simulink library "MotorControlLibrary"  (R2025b)
settings: Solver=VariableStepAuto  StartTime=0.0  StopTime=10.0  RelTol=1e-3
libraries: $bdroot x5
settings Model: Creator=tka008729  LastModifiedBy=tka008729

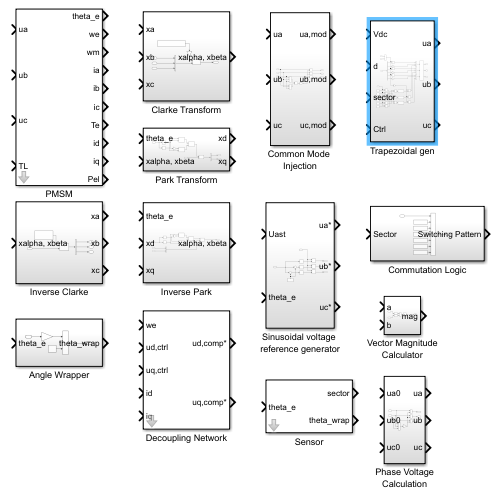
[thumbnail: Simulink's stored preview of the top-level diagram]
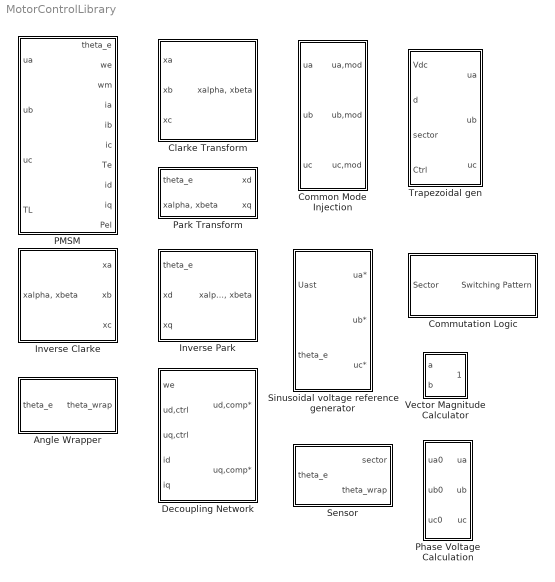
== system MotorControlLibrary ==
  Angle Wrapper : Subsystem
  Clarke Transform : Subsystem
  Common Mode Injection : Subsystem
  Commutation Logic : Subsystem
  Decoupling Network : Subsystem  mask(FOC Decoupling Network){Ls=0.000018, psi_PM=0.0021653734}
      mask prompts: Ls "Direct- and quadrute-axis inductances [Ls]"; psi_PM "Permanent magnet flux linkage [psi_PM]"
      mask help: Decouples direct- and quadrute-axis voltage components from eachother. Uses feedforward compensation. Relevant at higher speeds.
  Inverse Clarke : Subsystem
  Inverse Park : Subsystem
  PMSM : Subsystem  mask(PMSM){Rs=0.02125, Ls=0.000018, psi_PM=0.0021653734, p=14, J=0.0011, B=0.001}
      mask prompts: Rs "Phase resistance [Rs]"; Ls "Direct- and  quadrature-axis inductances [Ls]"; psi_PM "Permanent magnet flux linkage [psi_PM]"; p "Pole pairs [p]"; J "Moment of inertia [J]"; B "viscous friction coefficient [B]"
      mask help: Mathematical model of a non-salient permanent magnet synchronous motor (PMSM).
  Park Transform : Subsystem
  Phase Voltage Calculation : Subsystem
  Sensor : Subsystem  mask(Sector Sensor){phi_e=0}
      mask prompts: phi_e "Electrical angle offset [phi_e]"
      mask help: Converts continueous electrical angle in six-step control sector information.
  Sinusoidal voltage reference generator : Subsystem
  Trapezoidal gen : Subsystem
  Vector Magnitude Calculator : Subsystem

== system MotorControlLibrary/Angle Wrapper ==
  theta_e : Inport
  Constant : Constant  Value=360
  Gain6 : Gain  Gain=180/pi
  Math Function : Math  Operator=mod
  theta_wrap : Outport
  wires:
  Constant/1 -> Math Function/2
  Gain6/1 -> Math Function/1  "theta_deg"
  theta_e/1 -> Gain6/1
  Math Function/1 -> theta_wrap/1  "theta_wrap"

== system MotorControlLibrary/Clarke Transform ==
  xa : Inport
  xb : Inport  Port=2
  xc : Inport  Port=3
  Constant : Constant  Value=[1 -1/2 -1/2; 0 sqrt(3)/2 -sqrt(3)/2]
  Gain2 : Gain  Gain=2/3
  Mux : Mux  Inputs=3
  Product : Product  Multiplication=Matrix(*)
  "xalpha, xbeta" : Outport
  wires:
  xa/1 -> Mux/1
  xc/1 -> Mux/3
  Product/1 -> "xalpha, xbeta"/1
  Mux/1 -> Product/2
  Constant/1 -> Gain2/1
  xb/1 -> Mux/2
  Gain2/1 -> Product/1

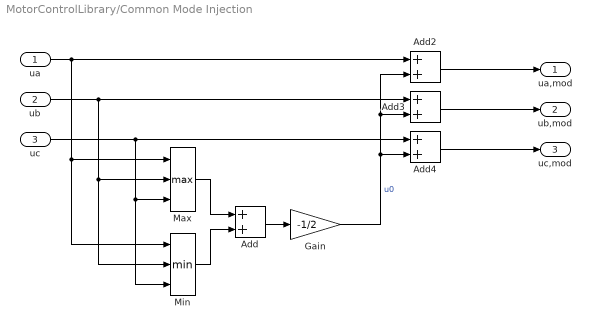
== system MotorControlLibrary/Common Mode Injection ==
  ua : Inport
  ub : Inport  Port=2
  uc : Inport  Port=3
  Add{,2..4} (4 alike) : Sum
  Gain : Gain  Gain=-1/2
  Max : MinMax  Function=max  Inputs=3
  Min : MinMax  Inputs=3
  ua,mod : Outport
  ub,mod : Outport  Port=2
  uc,mod : Outport  Port=3
  wires:
  Add2/1 -> ua,mod/1
  Add3/1 -> ub,mod/1
  Min/1 -> Add/2
  Add4/1 -> uc,mod/1
  Add/1 -> Gain/1
  Gain/1 -> Add2/2, Add3/2, Add4/2  "u0"
  ub/1 -> Max/2, Min/2, Add3/1
  Max/1 -> Add/1
  uc/1 -> Max/3, Min/3, Add4/1
  ua/1 -> Min/1, Max/1, Add2/1

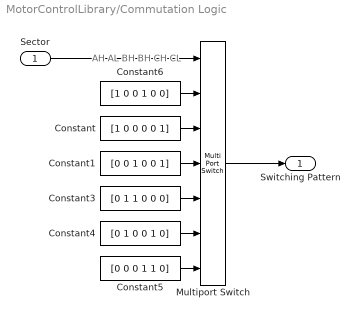
== system MotorControlLibrary/Commutation Logic ==
  note: AH AL BH BH CH CL
  Sector : Inport
  Constant : Constant  Value=[1 0 0 0 0 1]
  Constant1 : Constant  Value=[0 0 1 0 0 1]
  Constant3 : Constant  Value=[0 1 1 0 0 0]
  Constant4 : Constant  Value=[0 1 0 0 1 0]
  Constant5 : Constant  Value=[0 0 0 1 1 0]
  Constant6 : Constant  Value=[1 0 0 1 0 0]
  Multiport Switch : MultiPortSwitch  Inputs=6  DiagnosticForDefault=None  SaturateOnIntegerOverflow=off  InputSameDT=off
  Switching Pattern : Outport
  wires:
  Sector/1 -> Multiport Switch/1
  Multiport Switch/1 -> Switching Pattern/1
  Constant6/1 -> Multiport Switch/2
  Constant/1 -> Multiport Switch/3
  Constant1/1 -> Multiport Switch/4
  Constant3/1 -> Multiport Switch/5
  Constant5/1 -> Multiport Switch/7
  Constant4/1 -> Multiport Switch/6

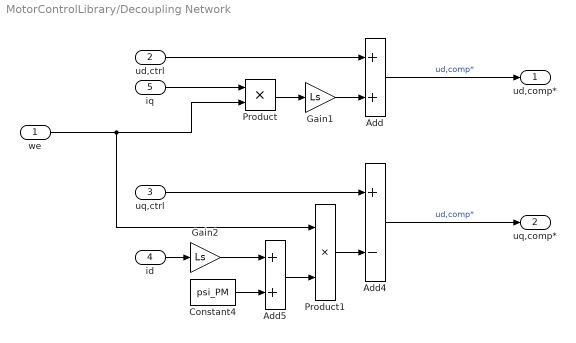
== system MotorControlLibrary/Decoupling Network ==
  we : Inport
  ud,ctrl : Inport  Port=2
  uq,ctrl : Inport  Port=3
  id : Inport  Port=4
  iq : Inport  Port=5
  Add : Sum
  Add4 : Sum  Inputs=+-
  Add5 : Sum
  Constant4 : Constant  Value=psi_PM
  Gain1 : Gain  Gain=Ls
  Gain2 : Gain  Gain=Ls
  Product : Product
  Product1 : Product
  ud,comp* : Outport
  uq,comp* : Outport  Port=2
  wires:
  iq/1 -> Product/1
  Product1/1 -> Add4/2
  Add5/1 -> Product1/2
  Constant4/1 -> Add5/2
  Gain2/1 -> Add5/1
  Add4/1 -> uq,comp*/1  "ud,comp*"
  Product/1 -> Gain1/1
  Gain1/1 -> Add/2
  ud,ctrl/1 -> Add/1
  id/1 -> Gain2/1
  Add/1 -> ud,comp*/1  "ud,comp*"
  we/1 -> Product1/1, Product/2
  uq,ctrl/1 -> Add4/1

== system MotorControlLibrary/Inverse Clarke ==
  "xalpha, xbeta" : Inport
  Constant1 : Constant  Value=[1 0; -1/2 sqrt(3)/2; -1/2 -sqrt(3)/2]
  Demux1 : Demux  Outputs=3
  Matrix Multiply : Product  Multiplication=Matrix(*)
  xa : Outport
  xb : Outport  Port=2
  xc : Outport  Port=3
  wires:
  Matrix Multiply/1 -> Demux1/1
  Constant1/1 -> Matrix Multiply/1
  Demux1/2 -> xb/1
  Demux1/3 -> xc/1
  Demux1/1 -> xa/1
  "xalpha, xbeta"/1 -> Matrix Multiply/2

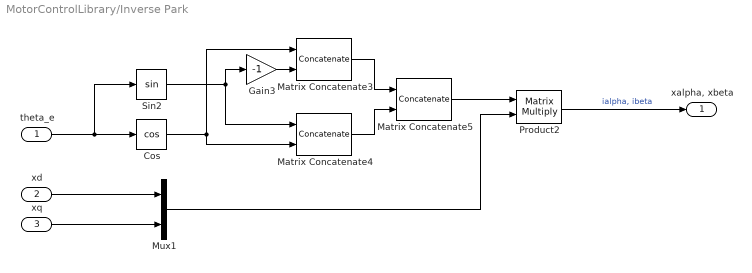
== system MotorControlLibrary/Inverse Park ==
  theta_e : Inport
  xd : Inport  Port=2
  xq : Inport  Port=3
  Cos : Trigonometry  Operator=cos
  Gain3 : Gain  Gain=-1
  Matrix Concatenate3 : Concatenate  Mode=Multidimensional array  ConcatenateDimension=2
  Matrix Concatenate4 : Concatenate  Mode=Multidimensional array  ConcatenateDimension=2
  Matrix Concatenate5 : Concatenate  Mode=Multidimensional array
  Mux1 : Mux  Inputs=2
  Product2 : Product  Multiplication=Matrix(*)
  Sin2 : Trigonometry
  "xalpha, xbeta" : Outport
  wires:
  theta_e/1 -> Sin2/1, Cos/1
  Gain3/1 -> Matrix Concatenate3/2
  Cos/1 -> Matrix Concatenate3/1, Matrix Concatenate4/2
  Mux1/1 -> Product2/2
  xq/1 -> Mux1/2
  Matrix Concatenate4/1 -> Matrix Concatenate5/2
  Matrix Concatenate5/1 -> Product2/1
  Product2/1 -> "xalpha, xbeta"/1  "ialpha, ibeta"
  Sin2/1 -> Matrix Concatenate4/1, Gain3/1
  Matrix Concatenate3/1 -> Matrix Concatenate5/1
  xd/1 -> Mux1/1

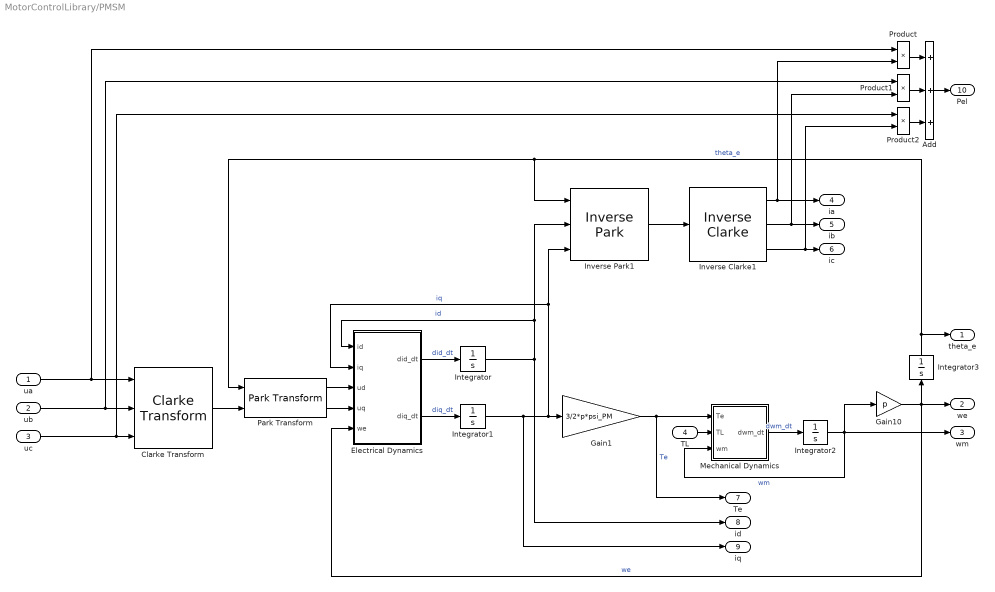
== system MotorControlLibrary/PMSM ==
  ua : Inport  Unit=V
  ub : Inport  Port=2  Unit=V
  uc : Inport  Port=3  Unit=V
  TL : Inport  Port=4
  Add : Sum  Inputs=+++
  Clarke Transform : $bdroot/Clarke Transform  SystemSampleTime=-1  VariantActivationTime=update diagram  EmptyChoice=off  PassThrough=off  PassThroughVariantControl=(default)  EmptyChoiceVariantControl=(default)  AllowFlexibleInterface=on  Latency=0  AutoFrameSizeCalculation=off
  Electrical Dynamics : Subsystem
  Gain1 : Gain  Gain=3/2*p*psi_PM
  Gain10 : Gain  Gain=p
  Integrator{,1..3} (4 alike) : Integrator
  Inverse Clarke1 : $bdroot/Inverse Clarke  SystemSampleTime=-1  VariantActivationTime=update diagram  EmptyChoice=off  PassThrough=off  PassThroughVariantControl=(default)  EmptyChoiceVariantControl=(default)  AllowFlexibleInterface=on  Latency=0  AutoFrameSizeCalculation=off
  Inverse Park1 : $bdroot/Inverse Park  SystemSampleTime=-1  VariantActivationTime=update diagram  EmptyChoice=off  PassThrough=off  PassThroughVariantControl=(default)  EmptyChoiceVariantControl=(default)  AllowFlexibleInterface=on  Latency=0  AutoFrameSizeCalculation=off
  Mechanical Dynamics : Subsystem
  Park Transform : $bdroot/Park Transform  SystemSampleTime=-1  VariantActivationTime=update diagram  EmptyChoice=off  PassThrough=off  PassThroughVariantControl=(default)  EmptyChoiceVariantControl=(default)  AllowFlexibleInterface=on  Latency=0  AutoFrameSizeCalculation=off
  Product : Product
  Product1 : Product
  Product2 : Product
  theta_e : Outport
  we : Outport  Port=2
  wm : Outport  Port=3
  ia : Outport  Port=4
  ib : Outport  Port=5
  ic : Outport  Port=6
  Te : Outport  Port=7
  id : Outport  Port=8
  iq : Outport  Port=9
  Pel : Outport  Port=10
  wires:
  Integrator3/1 -> Inverse Park1/1, Park Transform/1, theta_e/1  "theta_e"
  Gain10/1 -> Electrical Dynamics/5(we), Integrator3/1, we/1  "we"
  Integrator1/1 -> Inverse Park1/3, Electrical Dynamics/2(iq), Gain1/1, iq/1  "iq"
  Gain1/1 -> Te/1, Mechanical Dynamics/1(Te)  "Te"
  TL/1 -> Mechanical Dynamics/2(TL)
  Mechanical Dynamics/1(dwm_dt) -> Integrator2/1  "dwm_dt"
  Integrator2/1 -> Mechanical Dynamics/3(wm), Gain10/1, wm/1  "wm"
  Integrator/1 -> id/1, Inverse Park1/2, Electrical Dynamics/1(id)  "id"
  Electrical Dynamics/1(did_dt) -> Integrator/1  "did_dt"
  Electrical Dynamics/2(diq_dt) -> Integrator1/1  "diq_dt"
  Inverse Clarke1/2 -> ib/1, Product1/2
  Inverse Clarke1/1 -> ia/1, Product/2
  Inverse Clarke1/3 -> Product2/2, ic/1
  Clarke Transform/1 -> Park Transform/2
  Park Transform/1 -> Electrical Dynamics/3(ud)
  Park Transform/2 -> Electrical Dynamics/4(uq)
  ub/1 -> Product1/1, Clarke Transform/2
  ua/1 -> Product/1, Clarke Transform/1
  uc/1 -> Clarke Transform/3, Product2/1
  Inverse Park1/1 -> Inverse Clarke1/1
  Add/1 -> Pel/1
  Product1/1 -> Add/2
  Product/1 -> Add/1
  Product2/1 -> Add/3

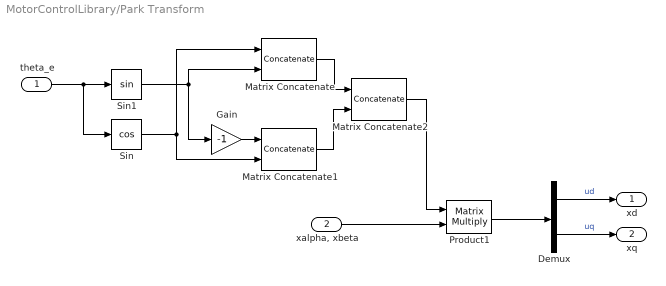
== system MotorControlLibrary/Park Transform ==
  theta_e : Inport
  "xalpha, xbeta" : Inport  Port=2
  Demux : Demux  Outputs=2
  Gain : Gain  Gain=-1
  Matrix Concatenate : Concatenate  Mode=Multidimensional array  ConcatenateDimension=2
  Matrix Concatenate1 : Concatenate  Mode=Multidimensional array  ConcatenateDimension=2
  Matrix Concatenate2 : Concatenate  Mode=Multidimensional array
  Product1 : Product  Multiplication=Matrix(*)
  Sin : Trigonometry  Operator=cos
  Sin1 : Trigonometry
  xd : Outport
  xq : Outport  Port=2
  wires:
  "xalpha, xbeta"/1 -> Product1/2
  Demux/1 -> xd/1  "ud"
  theta_e/1 -> Sin/1, Sin1/1
  Sin/1 -> Matrix Concatenate1/2, Matrix Concatenate/1
  Matrix Concatenate/1 -> Matrix Concatenate2/1
  Matrix Concatenate2/1 -> Product1/1
  Sin1/1 -> Matrix Concatenate/2, Gain/1
  Matrix Concatenate1/1 -> Matrix Concatenate2/2
  Gain/1 -> Matrix Concatenate1/1
  Product1/1 -> Demux/1
  Demux/2 -> xq/1  "uq"

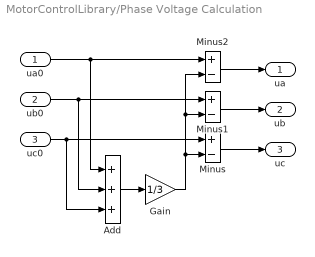
== system MotorControlLibrary/Phase Voltage Calculation ==
  ua0 : Inport
  ub0 : Inport  Port=2
  uc0 : Inport  Port=3
  Add : Sum  Inputs=+++
  Gain : Gain  Gain=1/3
  Minus : Sum  Inputs=+-
  Minus1 : Sum  Inputs=+-
  Minus2 : Sum  Inputs=+-
  ua : Outport
  ub : Outport  Port=2
  uc : Outport  Port=3
  wires:
  ub0/1 -> Minus1/1, Add/2
  Gain/1 -> Minus2/2, Minus1/2, Minus/2
  Minus1/1 -> ub/1
  uc0/1 -> Minus/1, Add/3
  ua0/1 -> Add/1, Minus2/1
  Minus/1 -> uc/1
  Add/1 -> Gain/1
  Minus2/1 -> ua/1

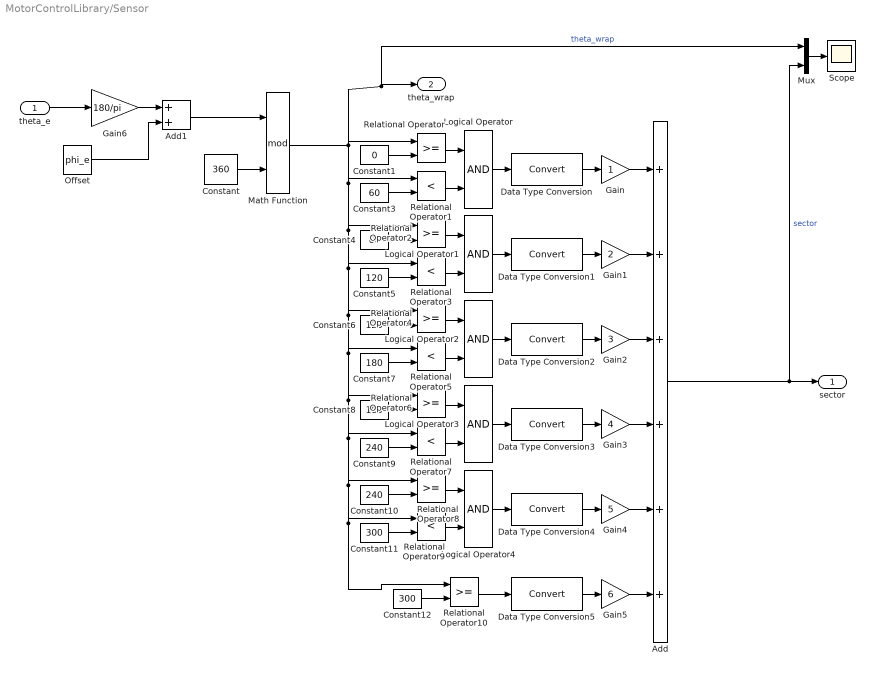
== system MotorControlLibrary/Sensor ==
  theta_e : Inport
  Add : Sum  Inputs=++++++
  Add1 : Sum
  Constant : Constant  Value=360
  Constant1 : Constant  Value=0
  Constant10 : Constant  Value=240
  Constant11 : Constant  Value=300
  Constant12 : Constant  Value=300
  Constant3 : Constant  Value=60
  Constant4 : Constant  Value=60
  Constant5 : Constant  Value=120
  Constant6 : Constant  Value=120
  Constant7 : Constant  Value=180
  Constant8 : Constant  Value=180
  Constant9 : Constant  Value=240
  Data Type Conversion{,1..5} (6 alike) : DataTypeConversion  SaturateOnIntegerOverflow=off  RndMeth=Floor
  Gain : Gain
  Gain1 : Gain  Gain=2
  Gain2 : Gain  Gain=3
  Gain3 : Gain  Gain=4
  Gain4 : Gain  Gain=5
  Gain5 : Gain  Gain=6
  Gain6 : Gain  Gain=180/pi
  Logical Operator{,1..4} (5 alike) : Logic  AllPortsSameDT=off  OutDataTypeStr=boolean
  Math Function : Math  Operator=mod
  Mux : Mux  Inputs=2
  Offset : Constant  Value=phi_e
  Relational Operator{,2,4,6,8,10} (6 alike) : RelationalOperator  OutDataTypeStr=boolean  RndMeth=Simplest  InputSameDT=off
  Relational Operator{1,3,5,7,9} (5 alike) : RelationalOperator  Operator=<  OutDataTypeStr=boolean  RndMeth=Simplest  InputSameDT=off
  Scope : Scope
      settings: ActiveDisplayYMinimum=-39.26586921535646  ActiveDisplayYMaximum=393.39282293820821  DataLoggingVariableName=ScopeData8
  sector : Outport
  theta_wrap : Outport  Port=2
  wires:
  Data Type Conversion2/1 -> Gain2/1
  Constant5/1 -> Relational Operator3/2
  Relational Operator6/1 -> Logical Operator3/1
  Gain5/1 -> Add/6
  Gain3/1 -> Add/4
  Data Type Conversion5/1 -> Gain5/1
  Relational Operator7/1 -> Logical Operator3/2
  Gain2/1 -> Add/3
  Constant10/1 -> Relational Operator8/2
  Relational Operator4/1 -> Logical Operator2/1
  Constant/1 -> Math Function/2
  Constant8/1 -> Relational Operator6/2
  Math Function/1 -> Mux/1, theta_wrap/1, Relational Operator/1, Relational Operator2/1, Relational Operator4/1, Relational Operator10/1, Relational Operator9/1, Relational Operator8/1, Relational Operator7/1, Relational Operator6/1, Relational Operator5/1, Relational Operator3/1, Relational Operator1/1  "theta_wrap"
  Constant12/1 -> Relational Operator10/2
  Constant6/1 -> Relational Operator4/2
  Relational Operator2/1 -> Logical Operator1/1
  Logical Operator2/1 -> Data Type Conversion2/1
  Data Type Conversion1/1 -> Gain1/1
  Relational Operator1/1 -> Logical Operator/2
  Constant11/1 -> Relational Operator9/2
  Add/1 -> Mux/2, sector/1  "sector"
  Logical Operator3/1 -> Data Type Conversion3/1
  Relational Operator5/1 -> Logical Operator2/2
  Relational Operator/1 -> Logical Operator/1
  Gain4/1 -> Add/5
  Logical Operator/1 -> Data Type Conversion/1
  Data Type Conversion3/1 -> Gain3/1
  Gain/1 -> Add/1
  Constant7/1 -> Relational Operator5/2
  Constant3/1 -> Relational Operator1/2
  Relational Operator9/1 -> Logical Operator4/2
  Constant9/1 -> Relational Operator7/2
  Constant4/1 -> Relational Operator2/2
  Logical Operator1/1 -> Data Type Conversion1/1
  Data Type Conversion4/1 -> Gain4/1
  Constant1/1 -> Relational Operator/2
  Logical Operator4/1 -> Data Type Conversion4/1
  Data Type Conversion/1 -> Gain/1
  Gain1/1 -> Add/2
  Relational Operator3/1 -> Logical Operator1/2
  Relational Operator8/1 -> Logical Operator4/1
  theta_e/1 -> Gain6/1
  Relational Operator10/1 -> Data Type Conversion5/1
  Gain6/1 -> Add1/1
  Add1/1 -> Math Function/1
  Offset/1 -> Add1/2
  Mux/1 -> Scope/1

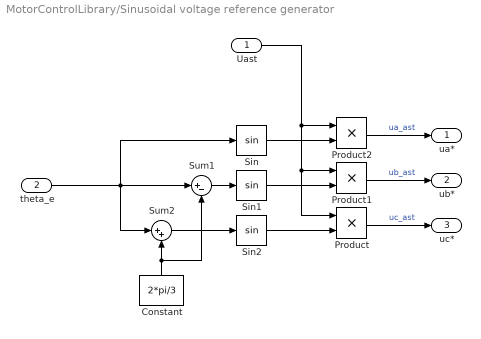
== system MotorControlLibrary/Sinusoidal voltage reference generator ==
  Uast : Inport
  theta_e : Inport  Port=2
  Constant : Constant  Value=2*pi/3
  Product : Product
  Product1 : Product
  Product2 : Product
  Sin : Trigonometry
  Sin1 : Trigonometry
  Sin2 : Trigonometry
  Sum1 : Sum  Inputs=|+-
  Sum2 : Sum  Inputs=|++
  ua* : Outport
  ub* : Outport  Port=2
  uc* : Outport  Port=3
  wires:
  Sum2/1 -> Sin2/1
  Product/1 -> uc*/1  "uc_ast"
  Sin1/1 -> Product1/2
  Constant/1 -> Sum2/2, Sum1/2
  Sum1/1 -> Sin1/1
  theta_e/1 -> Sin/1, Sum1/1, Sum2/1
  Sin2/1 -> Product/2
  Sin/1 -> Product2/2
  Product2/1 -> ua*/1  "ua_ast"
  Product1/1 -> ub*/1  "ub_ast"
  Uast/1 -> Product2/1, Product1/1, Product/1

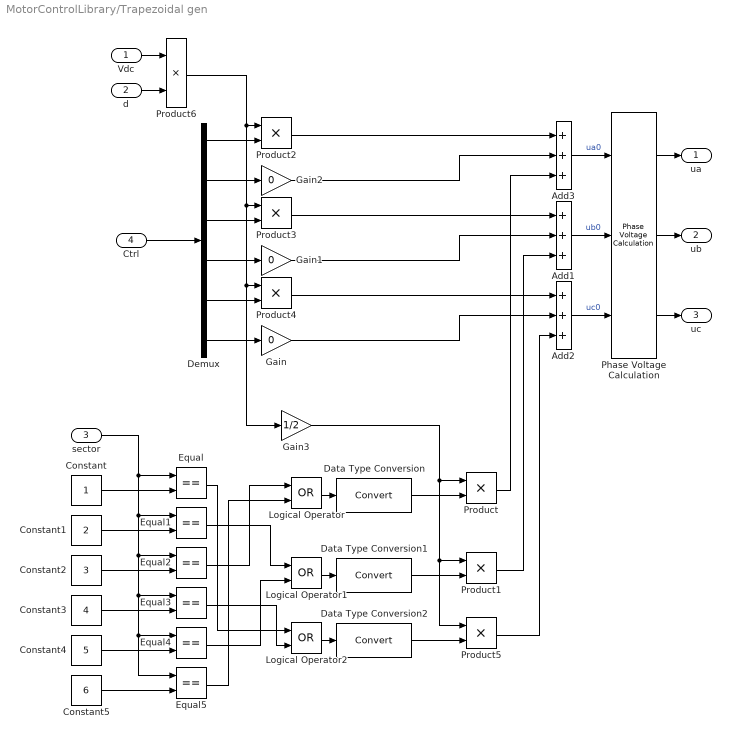
== system MotorControlLibrary/Trapezoidal gen ==
  Vdc : Inport
  d : Inport  Port=2
  sector : Inport  Port=3
  Ctrl : Inport  Port=4
  Add1 : Sum  Inputs=+++
  Add2 : Sum  Inputs=+++
  Add3 : Sum  Inputs=+++
  Constant : Constant
  Constant1 : Constant  Value=2
  Constant2 : Constant  Value=3
  Constant3 : Constant  Value=4
  Constant4 : Constant  Value=5
  Constant5 : Constant  Value=6
  Data Type Conversion : DataTypeConversion  SaturateOnIntegerOverflow=off  RndMeth=Floor
  Data Type Conversion1 : DataTypeConversion  SaturateOnIntegerOverflow=off  RndMeth=Floor
  Data Type Conversion2 : DataTypeConversion  SaturateOnIntegerOverflow=off  RndMeth=Floor
  Demux : Demux  Outputs=6
  Equal{,1..5} (6 alike) : RelationalOperator  Operator===  OutDataTypeStr=boolean  RndMeth=Simplest  InputSameDT=off
  Gain : Gain  Gain=0
  Gain1 : Gain  Gain=0
  Gain2 : Gain  Gain=0
  Gain3 : Gain  Gain=1/2
  Logical Operator : Logic  Operator=OR  AllPortsSameDT=off  OutDataTypeStr=boolean
  Logical Operator1 : Logic  Operator=OR  AllPortsSameDT=off  OutDataTypeStr=boolean
  Logical Operator2 : Logic  Operator=OR  AllPortsSameDT=off  OutDataTypeStr=boolean
  Phase Voltage Calculation : $bdroot/Phase Voltage Calculation  SystemSampleTime=-1  VariantActivationTime=update diagram  EmptyChoice=off  PassThrough=off  PassThroughVariantControl=(default)  EmptyChoiceVariantControl=(default)  AllowFlexibleInterface=on  Latency=0  AutoFrameSizeCalculation=off
  Product{,1..6} (7 alike) : Product
  ua : Outport
  ub : Outport  Port=2
  uc : Outport  Port=3
  wires:
  Demux/3 -> Product3/2
  Ctrl/1 -> Demux/1
  Demux/1 -> Product2/2
  Demux/5 -> Product4/2
  Product2/1 -> Add3/1
  Demux/6 -> Gain/1
  Demux/4 -> Gain1/1
  Demux/2 -> Gain2/1
  Gain2/1 -> Add3/2
  Data Type Conversion/1 -> Product/2
  Data Type Conversion1/1 -> Product1/2
  Data Type Conversion2/1 -> Product5/2
  Gain3/1 -> Product/1, Product1/1, Product5/1
  Product3/1 -> Add1/1
  Gain1/1 -> Add1/2
  Product4/1 -> Add2/1
  Gain/1 -> Add2/2
  Product/1 -> Add3/3
  Product1/1 -> Add1/3
  Product5/1 -> Add2/3
  sector/1 -> Equal5/1, Equal4/1, Equal3/1, Equal2/1, Equal1/1, Equal/1
  Constant/1 -> Equal/2
  Constant1/1 -> Equal1/2
  Constant2/1 -> Equal2/2
  Constant3/1 -> Equal3/2
  Constant4/1 -> Equal4/2
  Constant5/1 -> Equal5/2
  Logical Operator/1 -> Data Type Conversion/1
  Logical Operator1/1 -> Data Type Conversion1/1
  Logical Operator2/1 -> Data Type Conversion2/1
  Equal2/1 -> Logical Operator/1
  Equal5/1 -> Logical Operator/2
  Equal1/1 -> Logical Operator1/1
  Equal4/1 -> Logical Operator1/2
  Equal3/1 -> Logical Operator2/2
  Equal/1 -> Logical Operator2/1
  Product6/1 -> Gain3/1, Product4/1, Product3/1, Product2/1
  Vdc/1 -> Product6/1
  d/1 -> Product6/2
  Add1/1 -> Phase Voltage Calculation/2  "ub0"
  Phase Voltage Calculation/2 -> ub/1
  Add3/1 -> Phase Voltage Calculation/1  "ua0"
  Add2/1 -> Phase Voltage Calculation/3  "uc0"
  Phase Voltage Calculation/1 -> ua/1
  Phase Voltage Calculation/3 -> uc/1

== system MotorControlLibrary/Vector Magnitude Calculator ==
  a : Inport
  b : Inport  Port=2
  Add : Sum
  Square Root : Sqrt
  Square1 : Math  Operator=square
  Square2 : Math  Operator=square
  mag : Outport
  wires:
  Square2/1 -> Add/2
  a/1 -> Square1/1
  Square Root/1 -> mag/1  "c"
  Add/1 -> Square Root/1
  Square1/1 -> Add/1
  b/1 -> Square2/1

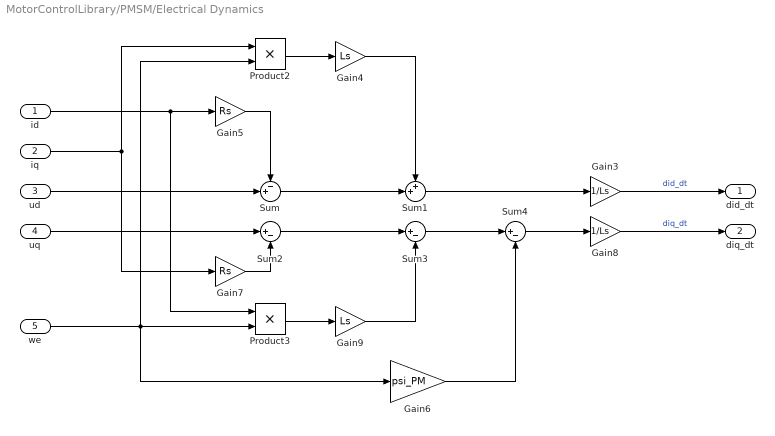
== system MotorControlLibrary/PMSM/Electrical Dynamics ==
  id : Inport
  iq : Inport  Port=2
  ud : Inport  Port=3
  uq : Inport  Port=4
  we : Inport  Port=5
  Gain3 : Gain  Gain=1/Ls
  Gain4 : Gain  Gain=Ls
  Gain5 : Gain  Gain=Rs
  Gain6 : Gain  Gain=psi_PM
  Gain7 : Gain  Gain=Rs
  Gain8 : Gain  Gain=1/Ls
  Gain9 : Gain  Gain=Ls
  Product2 : Product
  Product3 : Product
  Sum : Sum  Inputs=-+|
  Sum1 : Sum  Inputs=++|
  Sum2 : Sum  Inputs=|+-
  Sum3 : Sum  Inputs=|+-
  Sum4 : Sum  Inputs=|+-
  did_dt : Outport
  diq_dt : Outport  Port=2
  wires:
  Product2/1 -> Gain4/1
  Gain9/1 -> Sum3/2
  Gain7/1 -> Sum2/2
  Sum/1 -> Sum1/2
  iq/1 -> Gain7/1, Product2/1
  Product3/1 -> Gain9/1
  Sum4/1 -> Gain8/1
  ud/1 -> Sum/2
  Gain4/1 -> Sum1/1
  Gain6/1 -> Sum4/2
  Gain8/1 -> diq_dt/1  "diq_dt"
  Gain5/1 -> Sum/1
  id/1 -> Product3/1, Gain5/1
  uq/1 -> Sum2/1
  we/1 -> Product2/2, Gain6/1, Product3/2
  Sum3/1 -> Sum4/1
  Sum1/1 -> Gain3/1
  Gain3/1 -> did_dt/1  "did_dt"
  Sum2/1 -> Sum3/1

== system MotorControlLibrary/PMSM/Mechanical Dynamics ==
  Te : Inport
  TL : Inport  Port=2
  wm : Inport  Port=3
  Gain7 : Gain  Gain=1/J
  Gain9 : Gain  Gain=B
  Sum5 : Sum  Inputs=|+-
  Sum6 : Sum  Inputs=|+-
  dwm_dt : Outport
  wires:
  Gain9/1 -> Sum6/2
  TL/1 -> Sum5/2
  Te/1 -> Sum5/1
  Sum6/1 -> Gain7/1
  wm/1 -> Gain9/1
  Sum5/1 -> Sum6/1
  Gain7/1 -> dwm_dt/1  "dwm_dt"
